simulink model "PV_Math"  (R2020a)
settings: Solver=VariableStepAuto  StartTime=0.0  StopTime=10.0  RelTol=1e-3
libraries: simulink x3
settings Model: Creator=royde  LastModifiedBy=royde

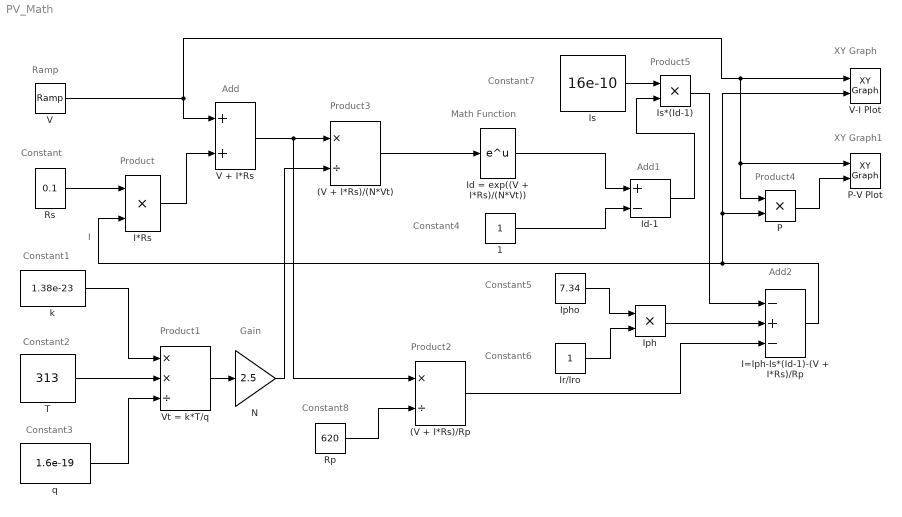
== system PV_Math ==
  note: Ramp
  note: I
  note: Constant
  note: Constant1
  note: Constant2
  note: Constant3
  note: Constant8
  note: Constant5
  note: Constant6
  note: Constant4
  note: Constant7
  note: Add
  note: Add1
  note: Add2
  note: Gain
  note: Product2
  note: Product1
  note: Product
  note: Product3
  note: Product5
  note: Product4
  note: Math Function
  note: XY Graph
  note: XY Graph1
  (V + I*Rs)/(N*Vt) : Product  Inputs=*/
  (V + I*Rs)/Rp : Product  Inputs=*/
  1 : Constant
  I*Rs : Product
  I=Iph-Is*(Id-1)-(V + I*Rs)/Rp : Sum  Inputs=-+-
  Id = exp((V + I*Rs)/(N*Vt)) : Math  SaturateOnIntegerOverflow=on
  Id-1 : Sum  Inputs=+-
  Iph : Product
  Ipho : Constant  Value=7.34
  Ir/Iro : Constant
  Is : Constant  Value=16e-10
  Is*(Id-1) : Product
  N : Gain  Gain=2.5
  P : Product
  P-V Plot : simulink/Sinks/XY Graph  xmin=0  xmax=1.5  ymin=0  ymax=6  st=-1
  Rp : Constant  Value=620
  Rs : Constant  Value=0.1
  T : Constant  Value=313
  V : simulink/Sources/Ramp  slope=1  start=0  InitialOutput=0
  V + I*Rs : Sum
  V-I Plot : simulink/Sinks/XY Graph  xmin=0  xmax=1.5  ymin=0  ymax=8  st=-1
  Vt = k*T/q : Product  Inputs=**/
  k : Constant  Value=1.38e-23
  q : Constant  Value=1.6e-19
  wires:
  Ipho/1 -> Iph/1
  Ir/Iro/1 -> Iph/2
  Rs/1 -> I*Rs/1
  I*Rs/1 -> V + I*Rs/2
  V + I*Rs/1 -> (V + I*Rs)/(N*Vt)/1, (V + I*Rs)/Rp/1
  k/1 -> Vt = k*T/q/1
  q/1 -> Vt = k*T/q/3
  T/1 -> Vt = k*T/q/2
  N/1 -> (V + I*Rs)/(N*Vt)/2
  (V + I*Rs)/(N*Vt)/1 -> Id = exp((V + I*Rs)/(N*Vt))/1
  Is/1 -> Is*(Id-1)/1
  Is*(Id-1)/1 -> I=Iph-Is*(Id-1)-(V + I*Rs)/Rp/1
  Iph/1 -> I=Iph-Is*(Id-1)-(V + I*Rs)/Rp/2
  Rp/1 -> (V + I*Rs)/Rp/2
  (V + I*Rs)/Rp/1 -> I=Iph-Is*(Id-1)-(V + I*Rs)/Rp/3
  I=Iph-Is*(Id-1)-(V + I*Rs)/Rp/1 -> P/2, V-I Plot/2, I*Rs/2
  P/1 -> P-V Plot/2
  V/1 -> V + I*Rs/1, P-V Plot/1, P/1, V-I Plot/1
  Id = exp((V + I*Rs)/(N*Vt))/1 -> Id-1/1
  Id-1/1 -> Is*(Id-1)/2
  1/1 -> Id-1/2
  Vt = k*T/q/1 -> N/1
